simulink model "car_model_FIXED"  (R2022b)
settings: Solver=VariableStepAuto  StartTime=0.0  StopTime=60  RelTol=1e-3
values from neighbouring files (symbols this model uses):
  ABS_MAX_TORQUE = [25 25 25 25]    [workspace.mat]
  ABS_MAX_TRQ_CMD = 50    [workspace.mat]
  ABS_MIN_TORQUE = [0.01 0.01 0.01 0.01]    [workspace.mat]
  acc_IC = 0    [workspace.mat]
  ACCELERATION_MAX = 30    [workspace.mat]
  ActSuspDutyCycle = 1    [workspace.mat]
  Aeq_left = [0.305756190204 0.308857786592 0.311945941182 0.315020811431 0.318082554689 0.321131328186 0.324167289011 0.327190594103 0.330201400225 0.333199863958 0.336186141681 0.339160389558 ... (261 elements, 1x261)]    [workspace.mat]
  Aeq_right = [-0.961664782545 -0.959835898365 -0.957982924115 -0.956106413788 -0.954206913862 -0.952284963337 -0.950341093764 -0.948375829284 -0.946389686656 -0.944383175301 -0.942356797333 -0.940311047601 ... (261 elements, 1x261)]    [workspace.mat]
  alpha_error = 0.1    [workspace.mat]
  ang_acc_hystersesis = 0.1    [workspace.mat]
  ang_IC = 0    [workspace.mat]
  ang_vel_IC = 0    [workspace.mat]
  area_air = 0.15    [workspace.mat]
  axb = -5    [workspace.mat]
  battery_current_IC = 0    [workspace.mat]
  BATTERY_CURRENT_MAX = 140    [workspace.mat]
  BATTERY_CURRENT_MIN = 0    [workspace.mat]
  battery_FT_IC = 300    [workspace.mat]
  battery_T_IC = 300    [workspace.mat]
  BATTERY_TEMPERATURE_MAX = 60    [workspace.mat]
  BATTERY_TEMPERATURE_MIN = 0    [workspace.mat]
  battery_voltage_IC = 332    [workspace.mat]
  BATTERY_VOLTAGE_MAX = 340    [workspace.mat]
  BATTERY_VOLTAGE_MIN = 60    [workspace.mat]
  br = 0.01    [workspace.mat]
  brake_bias = [0.35 0.35 0.15 0.15]    [workspace.mat]
  Brake_Pressure_IC = 1    [workspace.mat]
  ccl_IC = 0    [workspace.mat]
  CENTER_STEER_ANGLE_MAX = 130    [workspace.mat]
  covarience_matrix_IC = [0.001 0 0 0 0 0 0 0 0 0 0 0 ... (784 elements, 28x28)]    [workspace.mat]
  CURRENT_BUFFER = 25    [workspace.mat]
  cy_sweep = [13568.4166816 14020.2069783 14456.754831 14879.7402576 15289.7264712 15687.2766846 16072.954111 16447.3219632 16810.9434544 17164.3817975 17508.2002054 17842.9618912 ... (101 elements, 1x101)]    [workspace.mat]
  dB = 0.001    [workspace.mat]
  dcl_IC = 140    [workspace.mat]
  DCL_MAX = 130    [workspace.mat]
  DCL_MIN = 0    [workspace.mat]
  deadband_angle = 12    [workspace.mat]
  dIndex = 50    [workspace.mat]
  driver_t = 0.015    [workspace.mat]
  dt_OFF = 4.5    [workspace.mat]
  dt_ON = 7.5    [workspace.mat]
  dTx = 0.01    [workspace.mat]
  dx = 0.1    [workspace.mat]
  dZ = 0.295    [workspace.mat]
  efficiency_grid = [0.759500051293 0.787587791453 0.809832189108 0.826747821898 0.837164543102 0.842744381136 0.842258400104 0.838611650621 0.82826195101 0.814029316176 0.795690627225 0.7759791486 ... (2782 elements, 26x107)]    [workspace.mat]
  F0z = [0 0]    [workspace.mat]
  forward_look_straight = 5    [workspace.mat]
  forward_look_turn = 15    [workspace.mat]
  Fz_IC = 539.55    [workspace.mat]
  Fz_sweep = [200 210 220 230 240 250 260 270 280 290 300 310 ... (101 elements, 1x101)]    [workspace.mat]
  g = 9.81    [workspace.mat]
  GAIN_ABS = 100    [workspace.mat]
  gearbox_efficiency = [0.8 0.8 0.8 0.8]    [workspace.mat]
  gps_counter_IC = 0    [workspace.mat]
  gps_hz = 0.01    [workspace.mat]
  gr = [8.74786324786 8.74786324786 8.74786324786 8.74786324786]    [workspace.mat]
  I = 0    [workspace.mat]
  I_Driver = 1    [workspace.mat]
  indicies = [3 3.5 4 0.5 1 1.5 2 2.5 3 3.5 4 0.5 ... (27 elements, 1x27)]    [workspace.mat]
  IYY = 0.3    [workspace.mat]
  kx_sweep = [8779.958 9178.302 9576.646 9974.99 10373.334 10771.678 11170.022 11568.366 11966.71 12365.054 12763.398 13161.742 ... (101 elements, 1x101)]    [workspace.mat]
  l = [0.772 0.772]    [workspace.mat]
  lambda_star = 0.15    [workspace.mat]
  low_V_SA = 0.001    [workspace.mat]
  lr = 35    [workspace.mat]
  m_all = 220    [workspace.mat]
  m_body = 180    [workspace.mat]
  m_unsprung = [6 6 14 14]    [workspace.mat]
  MAG_MAX = 200    [workspace.mat]
  Max_Brake_Pressure = 100000000    [workspace.mat]
  Max_Driver_Input = 1    [workspace.mat]
  MAX_DTHETA_DRIVER = 360    [workspace.mat]
  MAX_I_Driver = 1    [workspace.mat]
  MAX_STEERING_ADJUST = 15    [workspace.mat]
  max_yaw = [0.705271610162 0.928228152446 1.12280857731 1.14131008363 1.08727026041 1.01377803859 0.938114723816 0.8718206875 0.815009168116 0.767481919497 0.727119764215 0.694403589394 ... (15 elements, 1x15)]    [workspace.mat]
  Min_Brake_Pressure = 1    [workspace.mat]
  Min_Driver_Input = 0    [workspace.mat]
  min_velocity_regen = 1.4    [workspace.mat]
  motor_current_IC = 0    [workspace.mat]
  MOTOR_CURRENT_MAX = 70    [workspace.mat]
  MOTOR_CURRENT_MIN = 0    [workspace.mat]
  MOTOR_ENABLE = [0 0 1 1]    [workspace.mat]
  motor_FT_IC = 300    [workspace.mat]
  motor_T_IC = 300    [workspace.mat]
  MOTOR_TEMPERATURE_MAX = 100    [workspace.mat]
  MOTOR_TEMPERATURE_MIN = 0    [workspace.mat]
  motor_voltage_IC = 332    [workspace.mat]
  MOTOR_VOLTAGE_MAX = 340    [workspace.mat]
  MOTOR_VOLTAGE_MIN = 90    [workspace.mat]
  motorControllerCurve = [25  260; 50  130; 75  0]    [workspace.mat]
  motorTempCurve = [140 138.6 134.4 127.4 117.6 105 89.6 71.4 50.4 26.6 0]    [workspace.mat]
  motorTempX = [75 77 79 81 83 85 87 89 91 93 95]    [workspace.mat]
  mu_star = 0.5    [workspace.mat]
  mx_sweep = [3.38348 3.3655067 3.3477908 3.3303323 3.3131312 3.2961875 3.2795012 3.2630723 3.2469008 3.2309867 3.21533 3.1999307 ... (101 elements, 1x101)]    [workspace.mat]
  my_sweep = [3.036232 3.015241699 2.994987032 2.975452753 2.956623616 2.938484375 2.921019784 2.904214597 2.888053568 2.872521451 2.857603 2.843282969 ... (101 elements, 1x101)]    [workspace.mat]
  noise_state = [1e-06 1e-06 1e-06 1e-06 0.005 0.005 0.005 1e-06 1e-06 1e-06 1e-06 1e-06 ... (28 elements, 28x1)]    [workspace.mat]
  omega_IC = 0    [workspace.mat]
  OMEGA_MAX = 150    [workspace.mat]
  OMEGA_MIN = 0    [workspace.mat]
  ORIENTATION_MAX = 360    [workspace.mat]
  P = 2    [workspace.mat]
  P_Driver = 0.7    [workspace.mat]
  P_High_Speed = 0.1    [workspace.mat]
  P_Steering_Adjust = 2    [workspace.mat]
  P_Straight_Adjust = 5    [workspace.mat]
  pos_IC = 0    [workspace.mat]
  POS_MAX = 300    [workspace.mat]
  q_thresh = 0.3    [workspace.mat]
  RE = 0.223    [workspace.mat]
  rho = 1.225    [workspace.mat]
  s = [0.649 0.621]    [workspace.mat]
  selected_maxvm = [49.86390724 16.21289794 8.219813569 8.05215527 7.103352929 8.35634983 13.87515039 8.72402841 22.75224945 36.67909339 19.32001297 25.09036962 ... (63 elements, 21x3)]    [workspace.mat]
  selected_sweep = [3 3 3 3 3 3 3 3 3 3 3 3 ... (1288 elements, 644x2)]    [workspace.mat]
  selected_track = [inf inf inf inf inf inf inf inf inf inf inf inf ... (37971 elements, 4219x9)]    [workspace.mat]
  shock_length_IC = 0.1    [workspace.mat]
  SHOCK_LENGTH_MAX = 0.25    [workspace.mat]
  SHOCK_LENGTH_MIN = 0    [workspace.mat]
  state_IC = [1 0 0 0 0 0 0 0 0 0 0 0 ... (28 elements, 28x1)]    [workspace.mat]
  steering_sweep = [0 5 10 15 20 25 30 35 40 45 50 55 ... (27 elements, 1x27)]    [workspace.mat]
  steering_Up_Grid = [0.551231966244 8.36038106007 16.1333806643 23.9559539118 31.8240691982 39.7561724339 47.7157531433 55.7845698794 64.1341708168 73.0798046026 82.7903081349 93.1297322155 ... (615 elements, 41x15)]    [workspace.mat]
  ... (+25 more)
undefined symbols (not defined in the file or in its folder): ax, ay, az, covA, covG, covM, covP, covV, DiscIntNeverNeededParam, fusion_t, fusion_t_sim, gps_ratio, IMU_accel, IMU_gyro, imu_hz, IMU_mag, location_lla_IC, p, phi, psi, q, r, sus, theta, trn, veh, VEH, whl, X, Xdot, Y, Ydot, Z, Zdot
libraries: fl_lib x82, nesl_utility x32, vehdynlibtire x10, vehdynlibsuspension x8, simulink x5, autolibutils x5, sharedtransform x5, sdl_lib x4, EngineCoolingComponents_lib x4, slpidlib x3, SimscapeFluids_lib x3, shared6dof x2
(part 2 of 14)

== system car_model_FIXED/Driver & Environment/Longitudinal Control ==
  Controller Information : Inport
  Sweep Information : Inport  Port=2
  AAS : Subsystem
  ABS : Subsystem
      settings: PortSchema="{\"entries\":[{\"content\":{\"sides\":[{\"content\":{\"connectorIds\":[\"In1\",\"In2\"]},\"type\":\"ConnectorPlacement.EquallySpacedRectSide\",\"uuid\":\"05691032-3f39-4834-938a-125b9d9c5bbe\"},{\"content\":{\"connectorIds\":[\"In3\",\"Out1\",\"Out2\"],\"side\":\"RIGHT\"},\"type\":\"ConnectorPlacement.EquallySpacedRectSide\",\"uuid\":\"b6342b01-7e0e-4c31-ae65-daa263149cd6\"},{\"content\":{\"connectorIds\":[],\"side\":\"TOP\"},\"type\":\"ConnectorPlacement.EquallySpacedRectSide\",\"uuid\":\"252d477f-1200-4151-9883-b9a128e2c38a\"}]},\"type\":\"ConnectorPlacement.EquallySpacedConnector\",\"uuid\":\"d67aaf26-3760-4411-918f-de910c7b3ed9\"}],\"packageUris\":[\"http://schema.mathworks.com/mf0/Connector/R2020b\"],\"version\":\"1.0\"}"
  AND : Logic  IconShape=distinctive  AllPortsSameDT=off  OutDataTypeStr=boolean
  Bus Selector : BusSelector  OutputSignals=v_cog,omega,v_error
  Bus Selector1 : BusSelector  OutputSignals=Velocity Error
  Constant5 : Constant  Value=YAW_ENABLE
  Constant6 : Constant  Value=0
  Less Than1 : RelationalOperator  Operator=<=  OutDataTypeStr=boolean  RndMeth=Simplest  InputSameDT=off
  Less Than2 : RelationalOperator  Operator=<  OutDataTypeStr=boolean  RndMeth=Simplest  InputSameDT=off
  NOT : Logic  Operator=NOT  IconShape=distinctive  AllPortsSameDT=off  OutDataTypeStr=boolean
  Product1 : Product  Inputs=3
  Product2 : Product  Inputs=3
  Saturation2 : Saturate  UpperLimit=Max_Brake_Pressure  LowerLimit=Min_Brake_Pressure
  Switch : Switch  Criteria=u2 > Threshold  SaturateOnIntegerOverflow=off  InputSameDT=off
  Switch1 : Switch  Criteria=u2 > Threshold  SaturateOnIntegerOverflow=off  InputSameDT=off
  Unit Delay{1,3..6} (5 alike) : UnitDelay  SampleTime=-1  HasFrameUpgradeWarning=on
  driver_input : Outport  PortDimensions=1
  brake_pedal : Outport  Port=2
  wires:
  Controller Information/1 -> Bus Selector/1
  Constant5/1 -> Switch/2, Product1/1, Switch1/2
  Sweep Information/1 -> Bus Selector1/1
  Bus Selector1/1 -> Switch1/3  "<Velocity Error>"
  Bus Selector/3 -> Unit Delay6/1, Switch1/1  "<v_error>"
  Bus Selector/1 -> Unit Delay3/1  "<v_cog>"
  Bus Selector/2 -> Unit Delay4/1  "<omega>"
  Product1/1 -> Saturation2/1
  Constant6/1 -> Less Than2/2, Less Than1/2
  AND/1 -> Unit Delay1/1, Product1/3
  ABS/1(Bx) -> Product1/2
  Less Than1/1 -> AND/1
  Less Than2/1 -> AND/2
  AAS/1(driver_input) -> Switch/3, Less Than1/1, Product2/3
  Saturation2/1 -> brake_pedal/1
  Switch1/1 -> Unit Delay5/1
  Product2/1 -> Switch/1
  Unit Delay1/1 -> NOT/1, ABS/3(ABS_ENABLE)
  NOT/1 -> Product2/1
  Unit Delay3/1 -> ABS/1(Vx)
  Unit Delay4/1 -> ABS/2(omega)
  Unit Delay5/1 -> AAS/1(v_error)
  Unit Delay6/1 -> Less Than2/1
  Switch/1 -> driver_input/1
  ABS/2(OFF_FLAG) -> Product2/2

== system car_model_FIXED/Driver & Environment/Reference Generator ==
  Analog Signals : Inport
  Driver Information : BusCreator  Inputs=12
  Memory : Memory  InitialCondition=1
  Memory1 : Memory  InitialCondition=1
  Reference Geneator : MATLAB Function  TreatAsAtomicUnit=on  SystemSampleTime=driver_t
  Selector : BusSelector  OutputSignals=psi,Vel,r,Disp,Omega
  Subsystem : Subsystem
  To Workspace : ToWorkspace  VariableName=Driver_Signals  SaveFormat=Timeseries  SampleTime=-1
  Unit Delay : UnitDelay  SampleTime=-1  HasFrameUpgradeWarning=on
  Unit Delay1 : UnitDelay  InitialCondition=1000  SampleTime=-1  HasFrameUpgradeWarning=on
  Controller Information : Outport
  wires:
  Analog Signals/1 -> To Workspace/1, Selector/1  "Driver"
  Selector/1 -> Subsystem/1(<psi>)  "<psi>"
  Reference Geneator/4(d_error) -> Driver Information/2
  Driver Information/1 -> Controller Information/1  "Driver Information"
  Selector/2 -> Reference Geneator/4(Vg)  "<Vel>"
  Reference Geneator/3(v_error) -> Driver Information/1
  Reference Geneator/6(v_cog) -> Driver Information/4
  Subsystem/1(psi_rev) -> Reference Geneator/3(psi)
  Reference Geneator/5(psi_error) -> Driver Information/3
  Reference Geneator/2(index_all) -> Memory/1
  Memory/1 -> Reference Geneator/2("index_all ")
  Reference Geneator/7(r_ref) -> Driver Information/5
  Reference Geneator/8(r_error) -> Driver Information/6
  Reference Geneator/15(ahead) -> Unit Delay/1
  Unit Delay/1 -> Reference Geneator/8("ahead ")
  Reference Geneator/12(omega) -> Driver Information/10
  Reference Geneator/9(x_ref) -> Driver Information/7
  Reference Geneator/10(y_ref) -> Driver Information/8
  Selector/3 -> Reference Geneator/5(yaw)  "<r>"
  Selector/4 -> Reference Geneator/6(pos)  "<Disp>"
  Reference Geneator/11(yaw_ref) -> Driver Information/9
  Memory1/1 -> Reference Geneator/1("index_small ")
  Reference Geneator/1(index_small) -> Memory1/1
  Reference Geneator/16(di_now) -> Unit Delay1/1
  Unit Delay1/1 -> Reference Geneator/9(di_prev)
  Selector/5 -> Reference Geneator/7("omega ")  "<Omega>"
  Reference Geneator/13(p_error) -> Driver Information/11
  Reference Geneator/14(Vnow) -> Driver Information/12

== system car_model_FIXED/Driver & Environment/Sweep Generator ==
  Analog Signals : Inport
  Bus Creator : BusCreator  Inputs=2
  Bus Selector : BusSelector  OutputSignals=Vel
  Memory : Memory  InitialCondition=1
  Sweep Generator : MATLAB Function  TreatAsAtomicUnit=on  SystemSampleTime=driver_t
  To Workspace : ToWorkspace  VariableName=counter  SaveFormat=Timeseries  SampleTime=-1
  Unit Delay : UnitDelay  SampleTime=-1  HasFrameUpgradeWarning=on
  Unit Delay1 : UnitDelay  InitialCondition=1  SampleTime=-1  HasFrameUpgradeWarning=on
  Controller Information : Outport
  wires:
  Analog Signals/1 -> Bus Selector/1
  Sweep Generator/2(vel_err) -> Bus Creator/1  "Velocity Error"
  Sweep Generator/3(ref_steer) -> Bus Creator/2  "Steering Angle"
  Bus Creator/1 -> Controller Information/1
  Bus Selector/1 -> Sweep Generator/2(vel)  "<Vel>"
  Sweep Generator/1(index) -> Memory/1
  Memory/1 -> Sweep Generator/1("index ")
  Sweep Generator/5(counter) -> Unit Delay/1, To Workspace/1
  Unit Delay/1 -> Sweep Generator/4("counter ")
  Sweep Generator/4(ON) -> Unit Delay1/1
  Unit Delay1/1 -> Sweep Generator/3("ON ")

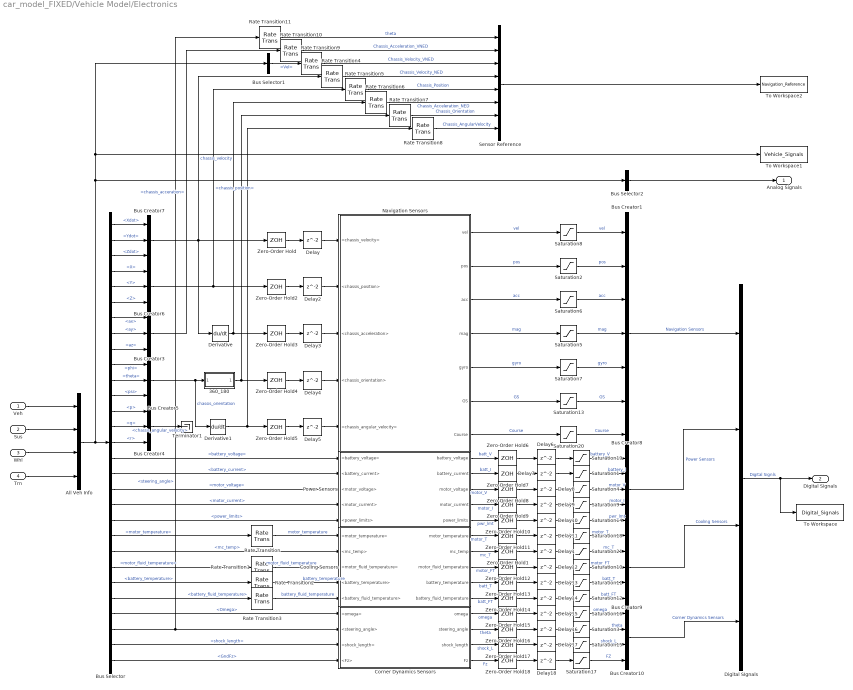
== system car_model_FIXED/Vehicle Model/Electronics ==
  Veh : Inport
  Sus : Inport  Port=2
  Whl : Inport  Port=3
  Trn : Inport  Port=4
  360_180 : Subsystem
  All Veh Info : BusCreator  Inputs=veh,sus,whl,trn
  Bus Creator1 : BusCreator  Inputs=7
  Bus Creator10 : BusCreator  Inputs=4
  Bus Creator3 : BusCreator  Inputs=ax,ay,az
  Bus Creator4 : BusCreator  Inputs=p,q,r
  Bus Creator5 : BusCreator  Inputs=phi,theta,psi
  Bus Creator6 : BusCreator  Inputs=X,Y,Z
  Bus Creator7 : BusCreator  Inputs=Xdot,Ydot,Zdot
  Bus Creator8 : BusCreator  Inputs=5
  Bus Creator9 : BusCreator  Inputs=5
  Bus Selector : BusSelector  OutputSignals=veh.InertFrm.Cg.Vel.Xdot,veh.InertFrm.Cg.Vel.Ydot,veh.InertFrm.Cg.Vel.Zdot,veh.InertFrm.Cg.Disp.X,veh.InertFrm.Cg.Disp.Y,veh.InertFrm.Cg.Disp.Z,veh.BdyFrm.Cg.Acc.ax,veh.BdyFrm.Cg.Acc.ay,veh.BdyFrm.Cg.Acc.az,veh.InertFrm.Cg.Ang.phi,veh.InertFrm.Cg.Ang.theta,veh.InertFrm.Cg.Ang.psi,veh.BdyFrm.Cg.AngVel.p,veh.BdyFrm.Cg.AngVel.q,veh.BdyFrm.Cg.AngVel.r,trn.battery_voltage,trn.battery_current,trn.motor_voltage,trn.motor_current,trn.power_limits,trn.motor_temperature,trn.mc_temp,trn.motor_fluid_temperature,trn.battery_temperature,trn.battery_fluid_temperature,whl.TireFrame.Omega,sus.Sus.steering_angle,sus.Sus.shock_length,whl.TireFrame.GndFz
  Bus Selector1 : BusSelector  OutputSignals=veh.BdyFrm.Cg.Vel
  Bus Selector2 : BusSelector  OutputSignals=veh.InertFrm.Cg.Disp,veh.InertFrm.Cg.Ang.psi,veh.BdyFrm.Cg.Vel,veh.BdyFrm.Cg.AngVel.r,sus.Sus.steering_angle,whl.TireFrame.Omega  OutputAsBus=on
  Cooling Sensors : Subsystem
  Corner Dynamics Sensors : Subsystem
  Delay : Delay  InitialCondition=([1;1]*vel_IC)'
  Delay1 : Delay  InitialCondition=[1 1; 1 1; 1 1; 1 1].*motor_T_IC
  Delay10 : Delay  InitialCondition=[dcl_IC; ccl_IC]*[1 1]
  Delay11 : Delay  InitialCondition=[1 1; 1 1; 1 1; 1 1].*motor_T_IC
  Delay12 : Delay  InitialCondition=[1 1; 1 1].*motor_FT_IC
  Delay13 : Delay  InitialCondition=[1 1].*battery_T_IC
  Delay14 : Delay  InitialCondition=[1 1].*battery_FT_IC
  Delay15 : Delay  InitialCondition=ones(1, 4, 2).*omega_IC
  Delay16 : Delay  InitialCondition=[1 1].*theta_IC
  Delay17 : Delay  InitialCondition=[1 1; 1 1; 1 1; 1 1].*shock_length_IC
  Delay18 : Delay  InitialCondition=[1 1; 1 1; 1 1; 1 1].*Fz_IC
  Delay2 : Delay  InitialCondition=[1 1; 1 1; 1 1].*pos_IC
  Delay3 : Delay  InitialCondition=[1 1; 1 1; 1 1].*acc_IC
  Delay4 : Delay  InitialCondition=[1 1; 1 1; 1 1].*ang_IC
  Delay5 : Delay  InitialCondition=[1 1; 1 1; 1 1].*ang_vel_IC
  Delay6 : Delay  InitialCondition=[1 1].*battery_voltage_IC
  Delay7 : Delay  InitialCondition=[1 1].*battery_current_IC
  Delay8 : Delay  InitialCondition=[1 1; 1 1; 1 1; 1 1].*motor_voltage_IC
  Delay9 : Delay  InitialCondition=ones(1, 4, 2).*motor_current_IC
  Derivative : Derivative
  Derivative1 : Derivative
  Digital SIgnals : BusCreator  Inputs=4
  Navigation Sensors : Subsystem
  Power Sensors : Subsystem
  Rate Transition : RateTransition  OutPortSampleTime=0
  Rate Transition1 : RateTransition  InitialCondition=[1 1].*motor_FT_IC  OutPortSampleTime=0
  Rate Transition{4..11} (8 alike) : RateTransition  Deterministic=off  OutPortSampleTime=fusion_t
  Rate Transition2 : RateTransition  OutPortSampleTime=0
  Rate Transition3 : RateTransition  OutPortSampleTime=0
  Saturation1 : Saturate  UpperLimit=BATTERY_CURRENT_MAX  LowerLimit=BATTERY_CURRENT_MIN
  Saturation10 : Saturate  UpperLimit=MOTOR_TEMPERATURE_MAX  LowerLimit=MOTOR_TEMPERATURE_MIN
  Saturation11 : Saturate  UpperLimit=BATTERY_TEMPERATURE_MAX  LowerLimit=BATTERY_TEMPERATURE_MIN
  Saturation12 : Saturate  UpperLimit=BATTERY_TEMPERATURE_MAX  LowerLimit=BATTERY_TEMPERATURE_MIN
  Saturation13 : Saturate  UpperLimit=VELOCITY_MAX  LowerLimit=-VELOCITY_MAX
  Saturation14 : Saturate  UpperLimit=DCL_MAX  LowerLimit=DCL_MIN
  Saturation15 : Saturate  UpperLimit=SHOCK_LENGTH_MAX  LowerLimit=SHOCK_LENGTH_MIN
  Saturation16 : Saturate  UpperLimit=OMEGA_MAX  LowerLimit=OMEGA_MIN
  Saturation17 : Saturate  UpperLimit=1200  LowerLimit=200
  Saturation18 : Saturate  UpperLimit=MOTOR_TEMPERATURE_MAX  LowerLimit=MOTOR_TEMPERATURE_MIN
  Saturation19 : Saturate  UpperLimit=BATTERY_VOLTAGE_MAX  LowerLimit=BATTERY_VOLTAGE_MIN
  Saturation2 : Saturate  UpperLimit=inf  LowerLimit=-inf
  Saturation20 : Saturate  UpperLimit=ORIENTATION_MAX  LowerLimit=-ORIENTATION_MAX
  Saturation21 : Saturate  UpperLimit=MOTOR_TEMPERATURE_MAX  LowerLimit=MOTOR_TEMPERATURE_MIN
  Saturation3 : Saturate  UpperLimit=CENTER_STEER_ANGLE_MAX  LowerLimit=-CENTER_STEER_ANGLE_MAX
  Saturation4 : Saturate  UpperLimit=MOTOR_VOLTAGE_MAX  LowerLimit=MOTOR_VOLTAGE_MIN
  Saturation5 : Saturate  UpperLimit=MAG_MAX  LowerLimit=-MAG_MAX
  Saturation6 : Saturate  UpperLimit=ACCELERATION_MAX  LowerLimit=-ACCELERATION_MAX
  Saturation7 : Saturate  UpperLimit=YAW_MAX  LowerLimit=-YAW_MAX
  Saturation8 : Saturate  UpperLimit=VELOCITY_MAX  LowerLimit=-VELOCITY_MAX
  Saturation9 : Saturate  UpperLimit=MOTOR_CURRENT_MAX  LowerLimit=MOTOR_CURRENT_MIN
  Sensor Reference : BusCreator  Inputs=8
  Terminator1 : Terminator
  To Workspace : ToWorkspace  VariableName=Digital_Signals  SaveFormat=Timeseries  SampleTime=-1
  To Workspace1 : ToWorkspace  VariableName=Vehicle_Signals  SaveFormat=Timeseries  SampleTime=-1
  To Workspace2 : ToWorkspace  VariableName=Navigation_Reference  SaveFormat=Timeseries  SampleTime=-1
  Zero-Order Hold : ZeroOrderHold  SampleTime=gps_hz
  Zero-Order Hold{1,6..18} (14 alike) : ZeroOrderHold  SampleTime=tvs_t_sim
  Zero-Order Hold2 : ZeroOrderHold  SampleTime=gps_hz
  Zero-Order Hold3 : ZeroOrderHold  SampleTime=imu_hz
  Zero-Order Hold4 : ZeroOrderHold  SampleTime=imu_hz
  Zero-Order Hold5 : ZeroOrderHold  SampleTime=imu_hz
  Analog Signals : Outport
  Digital Signals : Outport  Port=2
  wires:
  Sus/1 -> All Veh Info/2
  Whl/1 -> All Veh Info/3
  Veh/1 -> All Veh Info/1
  Trn/1 -> All Veh Info/4
  Bus Selector/7 -> Bus Creator3/1  "<ax>"
  Bus Selector/8 -> Bus Creator3/2  "<ay>"
  Bus Selector/9 -> Bus Creator3/3  "<az>"
  Bus Selector/13 -> Bus Creator4/1  "<p>"
  Bus Selector/14 -> Bus Creator4/2  "<q>"
  Bus Selector/15 -> Bus Creator4/3  "<r>"
  Bus Selector/1 -> Bus Creator7/1  "<Xdot>"
  Bus Selector/2 -> Bus Creator7/2  "<Ydot>"
  Bus Selector/10 -> Bus Creator5/1  "<phi>"
  Bus Selector/11 -> Bus Creator5/2  "<theta>"
  Bus Selector/12 -> Bus Creator5/3  "<psi>"
  Bus Selector/4 -> Bus Creator6/1  "<X>"
  Bus Selector/5 -> Bus Creator6/2  "<Y>"
  Bus Selector2/1 -> Analog Signals/1
  Bus Selector/3 -> Bus Creator7/3  "<Zdot>"
  Bus Selector/6 -> Bus Creator6/3  "<Z>"
  Bus Creator7/1 -> Zero-Order Hold/1, Rate Transition4/1, Derivative/1  "chassis_velocity"
  Bus Creator6/1 -> Zero-Order Hold2/1, Rate Transition5/1  "<chassis_position>"
  Bus Creator5/1 -> Derivative1/1, 360_180/1(<psi>)  "chassis_orientation"
  Bus Selector/20 -> Power Sensors/5(<power_limits>)  "<power_limits>"
  Bus Selector/17 -> Power Sensors/2(<battery_current>)  "<battery_current>"
  Bus Selector/19 -> Power Sensors/4(<motor_current>)  "<motor_current>"
  Bus Selector/18 -> Power Sensors/3(<motor_voltage>)  "<motor_voltage>"
  Bus Selector/21 -> Rate Transition/1  "<motor_temperature>"
  Bus Selector/26 -> Corner Dynamics Sensors/1(<omega>)  "<Omega>"
  Bus Selector/27 -> Corner Dynamics Sensors/2(<steering_angle>), Rate Transition11/1  "<steering_angle>"
  Bus Selector/28 -> Corner Dynamics Sensors/3(<shock_length>)  "<shock_length>"
  Bus Selector/29 -> Corner Dynamics Sensors/4(<Fz>)  "<GndFz>"
  Bus Selector/23 -> Rate Transition1/1  "<motor_fluid_temperature>"
  Bus Selector/16 -> Power Sensors/1(<battery_voltage>)  "<battery_voltage>"
  Bus Selector/24 -> Rate Transition2/1  "<battery_temperature>"
  Bus Selector/25 -> Rate Transition3/1  "<battery_fluid_temperature>"
  Navigation Sensors/1(vel) -> Saturation8/1  "vel"
  Navigation Sensors/2(pos) -> Saturation2/1  "pos"
  Navigation Sensors/3(acc) -> Saturation6/1  "acc"
  Navigation Sensors/4(mag) -> Saturation5/1  "mag"
  Navigation Sensors/5(gyro) -> Saturation7/1  "gyro"
  Power Sensors/1(battery_voltage) -> Zero-Order Hold6/1  "batt_V"
  Power Sensors/2(battery_current) -> Zero-Order Hold7/1  "batt_I"
  Power Sensors/3(motor_voltage) -> Zero-Order Hold8/1  "motor_V"
  Power Sensors/4(motor_current) -> Zero-Order Hold9/1  "motor_I"
  Power Sensors/5(power_limits) -> Zero-Order Hold10/1  "pwr_lmt"
  Cooling Sensors/1(motor_temperature) -> Zero-Order Hold11/1  "motor_T"
  Cooling Sensors/3(motor_fluid_temperature) -> Zero-Order Hold12/1  "motor_FT"
  Cooling Sensors/4(battery_temperature) -> Zero-Order Hold13/1  "batt_T"
  Cooling Sensors/5(battery_fluid_temperature) -> Zero-Order Hold14/1  "batt_FT"
  Corner Dynamics Sensors/1(omega) -> Zero-Order Hold15/1  "omega"
  Corner Dynamics Sensors/2(steering_angle) -> Zero-Order Hold16/1  "theta"
  Corner Dynamics Sensors/3(shock_length) -> Zero-Order Hold17/1  "shock_L"
  Corner Dynamics Sensors/4(Fz) -> Zero-Order Hold18/1  "Fz"
  Bus Creator1/1 -> Digital SIgnals/1  "Navigation Sensors"
  Bus Creator8/1 -> Digital SIgnals/2  "Power Sensors"
  Bus Creator10/1 -> Digital SIgnals/4  "Corner Dynamics Sensors"
  Digital SIgnals/1 -> Digital Signals/1, To Workspace/1  "Digital Signls"
  Saturation15/1 -> Bus Creator10/3  "shock_L"
  Saturation17/1 -> Bus Creator10/4  "FZ"
  Saturation3/1 -> Bus Creator10/2  "theta"
  Saturation16/1 -> Bus Creator10/1  "omega"
  Saturation8/1 -> Bus Creator1/1  "vel"
  Saturation2/1 -> Bus Creator1/2  "pos"
  Saturation6/1 -> Bus Creator1/3  "acc"
  Saturation5/1 -> Bus Creator1/4  "mag"
  Saturation7/1 -> Bus Creator1/5  "gyro"
  Saturation19/1 -> Bus Creator8/1  "battery_V"
  Saturation1/1 -> Bus Creator8/2  "battery_I"
  Saturation9/1 -> Bus Creator8/4  "motor_I"
  Saturation4/1 -> Bus Creator8/3  "motor_V"
  Saturation14/1 -> Bus Creator8/5  "pwr_lmt"
  Saturation18/1 -> Bus Creator9/1  "motor_T"
  Saturation10/1 -> Bus Creator9/3  "motor_FT"
  Saturation11/1 -> Bus Creator9/4  "batt_T"
  Saturation12/1 -> Bus Creator9/5  "batt_FT"
  Zero-Order Hold6/1 -> Delay6/1
  Zero-Order Hold7/1 -> Delay7/1
  Zero-Order Hold8/1 -> Delay8/1
  Zero-Order Hold9/1 -> Delay9/1
  Zero-Order Hold10/1 -> Delay10/1
  Zero-Order Hold11/1 -> Delay11/1
  Zero-Order Hold12/1 -> Delay12/1
  Zero-Order Hold13/1 -> Delay13/1
  Zero-Order Hold14/1 -> Delay14/1
  Zero-Order Hold15/1 -> Delay15/1
  Zero-Order Hold16/1 -> Delay16/1
  Zero-Order Hold17/1 -> Delay17/1
  Zero-Order Hold18/1 -> Delay18/1
  Delay6/1 -> Saturation19/1
  Delay7/1 -> Saturation1/1
  Delay8/1 -> Saturation4/1
  Delay9/1 -> Saturation9/1
  Delay10/1 -> Saturation14/1
  Delay11/1 -> Saturation18/1
  Delay12/1 -> Saturation10/1
  Delay13/1 -> Saturation11/1
  Delay14/1 -> Saturation12/1
  Delay15/1 -> Saturation16/1
  Delay16/1 -> Saturation3/1
  Delay17/1 -> Saturation15/1
  Delay18/1 -> Saturation17/1
  Rate Transition/1 -> Cooling Sensors/1(<motor_temperature>)  "motor_temperature"
  Rate Transition1/1 -> Cooling Sensors/3(<motor_fluid_temperature>)  "motor_fluid_temperature"
  Rate Transition2/1 -> Cooling Sensors/4(<battery_temperature>)  "battery_temperature"
  Rate Transition3/1 -> Cooling Sensors/5(<battery_fluid_temperature>)  "battery_fluid_temperature"
  Bus Creator9/1 -> Digital SIgnals/3  "Cooling Sensors"
  Navigation Sensors/6(GS) -> Saturation13/1  "GS"
  Navigation Sensors/7(Course) -> Saturation20/1  "Course"
  Saturation13/1 -> Bus Creator1/6  "GS"
  Saturation20/1 -> Bus Creator1/7  "Course"
  Delay/1 -> Navigation Sensors/1(<chassis_velocity>)
  Delay2/1 -> Navigation Sensors/2(<chassis_position>)
  Derivative/1 -> Zero-Order Hold3/1, Rate Transition6/1
  360_180/1(psi_rev) -> Zero-Order Hold4/1, Rate Transition7/1
  Delay3/1 -> Navigation Sensors/3(<chassis_acceleration>)
  Delay4/1 -> Navigation Sensors/4(<chassis_orientation>)
  Delay5/1 -> Navigation Sensors/5(<chassis_angular_velocity>)
  Derivative1/1 -> Zero-Order Hold5/1, Rate Transition8/1
  Sensor Reference/1 -> To Workspace2/1
  Rate Transition4/1 -> Sensor Reference/4  "Chassis_Velocity_NED"
  Rate Transition5/1 -> Sensor Reference/5  "Chassis_Position"
  Rate Transition6/1 -> Sensor Reference/6  "Chassis_Acceleration_NED"
  Rate Transition7/1 -> Sensor Reference/7  "Chassis_Orientation"
  Rate Transition8/1 -> Sensor Reference/8  "Chassis_AngularVelocity"
  Bus Creator4/1 -> Terminator1/1  "<chassis_angular_velocity>"
  Bus Creator3/1 -> Rate Transition10/1  "<chassis_acceration>"
  Zero-Order Hold/1 -> Delay/1
  Zero-Order Hold2/1 -> Delay2/1
  Zero-Order Hold3/1 -> Delay3/1
  Zero-Order Hold4/1 -> Delay4/1
  Zero-Order Hold5/1 -> Delay5/1
  Bus Selector/22 -> Cooling Sensors/2(<mc_temp>)  "<mc_temp>"
  Zero-Order Hold1/1 -> Delay1/1
  Delay1/1 -> Saturation21/1
  Cooling Sensors/2(mc_temp) -> Zero-Order Hold1/1  "mc_T"
  Saturation21/1 -> Bus Creator9/2  "mc_T"
  All Veh Info/1 -> Bus Selector1/1, To Workspace1/1, Bus Selector2/1, Bus Selector/1
  Bus Selector1/1 -> Rate Transition9/1  "<Vel>"
  Rate Transition9/1 -> Sensor Reference/3  "Chassis_Velocity_VNED"
  Rate Transition10/1 -> Sensor Reference/2  "Chassis_Acceleration_VNED"
  Rate Transition11/1 -> Sensor Reference/1  "theta"
